simulink model "LAB1_3_mot"  (R2024b)
settings: Solver=ode3  StartTime=0.0  StopTime=10  FixedStep=0.001  RelTol=1e-3
values from neighbouring files (symbols this model uses):
  delta_c = 1/sqrt(2)    [LAB1_Corretto.m]    (also in LAB1_GIOI.m)
  K_g = K_e(2:3)    [LAB1_Corretto.m]    (also in LAB1_GIOI.m)
  KI = K_e(1)    [LAB1_Corretto.m]    (also in LAB1_GIOI.m)
  Nu = N(3)    [LAB1_Corretto.m]    (also in LAB1_GIOI.m)
  Nx = N(1:2)    [LAB1_Corretto.m]    (also in LAB1_GIOI.m)
  w_c = 2*pi*50    (= 314.159265359)    [LAB1_Corretto.m]    (also in LAB1_GIOI.m)
undefined symbols (not defined in the file or in its folder): degs2rpm, den_Hi, den_Hw, mot, National_Instruments, num_Hi, num_Hw, PCI, rpm2rads, sens
libraries: sldrtlib x3
settings Model: SimulationMode=external  ExtModeTrigDuration=100001  Creator=delpratogi  LastModifiedBy=delpratogi
settings DataIOCC: ReturnWorkspaceOutputs=off
settings HardwareCC: ProdBitPerLong=64  ProdHWDeviceType=Intel->x86-64 (Linux 64)
settings RTWCC: Description=Simulink Desktop Real-Time  SystemTargetFile=sldrt.tlc  TemplateMakefile=sldrt.tmf  RTWCompilerOptimization=on
settings CodeAppCC: MaxIdLength=95
settings SimulinkDesktopRealTimeCC: TargetLibSuffix=_sldrt.a  TargetPreCompLibLocation=C:\Program Files\MATLAB\R2024b\toolbox\sldrt\lib\win64  ParMdlRefBuildCompliant=on

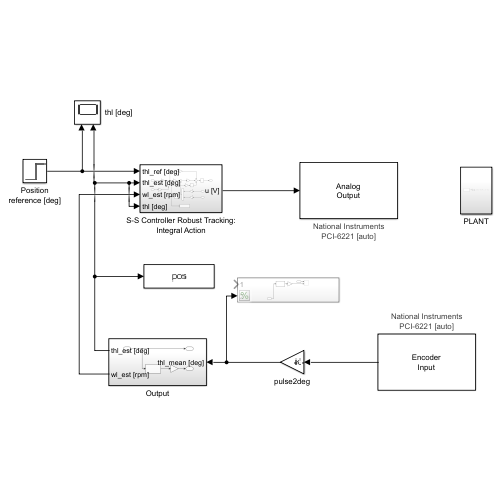
[thumbnail: Simulink's stored preview of the top-level diagram]
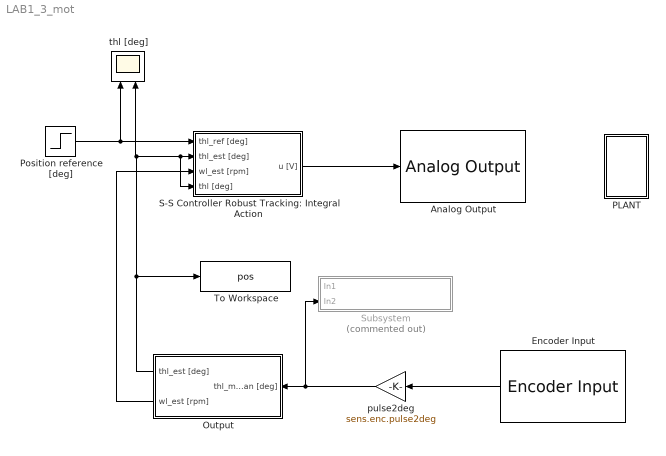
== system LAB1_3_mot ==
  Analog Output : sldrtlib/Analog Output  SampleTime=0.001  MaxMissedTicks=10  ShowMissedTicks=off  YieldWhenWaiting=off  DrvName=National_Instruments/PCI-6221  DrvAddress=4294967295  DrvOptions=[0 0 0 2 0]  Channels=1  RangeMode=1  VoltRange=1  InitialValue=0  FinalValue=0
      settings: AttributesFormatString=National Instruments\nPCI-6221 [auto]
  Encoder Input : sldrtlib/Encoder Input  SampleTime=0.001  MaxMissedTicks=10  ShowMissedTicks=off  YieldWhenWaiting=off  DrvName=National_Instruments/PCI-6221  DrvAddress=4294967295  DrvOptions=[0 0 0 2 0]  Channels=1  QuadMode=3  IndexPulse=1  InputFilter=Inf  DataType=1
      settings: AttributesFormatString=National Instruments\nPCI-6221 [auto]
  Output : Subsystem
  PLANT : Subsystem
  Position reference [deg] : Step  Time=0  After=120  SampleTime=0  ZeroCross=off
  S-S Controller Robust Tracking: Integral Action : Subsystem
  Subsystem : Subsystem  Commented=on
  To Workspace : ToWorkspace  VariableName=pos  SaveFormat=Structure With Time  SampleTime=-1
  pulse2deg : Gain  Gain=sens.enc.pulse2deg
  thl [deg] : Scope  NumInputPorts=2
  wires:
  Encoder Input/1 -> pulse2deg/1
  pulse2deg/1 -> Subsystem/2(In2), Output/1(thl_mean [deg])
  S-S Controller Robust Tracking: Integral Action/1(u [V]) -> Analog Output/1
  Output/2(wl_est [rpm]) -> S-S Controller Robust Tracking: Integral Action/3(wl_est [rpm])
  Position reference [deg]/1 -> S-S Controller Robust Tracking: Integral Action/1(thl_ref [deg]), thl [deg]/1
  Output/1(thl_est [deg]) -> S-S Controller Robust Tracking: Integral Action/4(thl [deg]), S-S Controller Robust Tracking: Integral Action/2(thl_est [deg]), thl [deg]/2, To Workspace/1

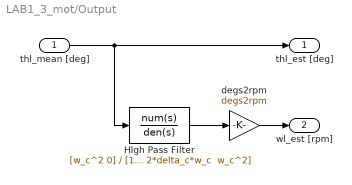
== system LAB1_3_mot/Output ==
  thl_mean [deg] : Inport
  HIgh Pass Filter : TransferFcn  Numerator=[w_c^2 0]  Denominator="[1 2*delta_c*w_c  w_c^2]"
  degs2rpm : Gain  Gain=degs2rpm
  thl_est [deg] : Outport
  wl_est [rpm] : Outport  Port=2
  wires:
  thl_mean [deg]/1 -> HIgh Pass Filter/1, thl_est [deg]/1
  HIgh Pass Filter/1 -> degs2rpm/1
  degs2rpm/1 -> wl_est [rpm]/1

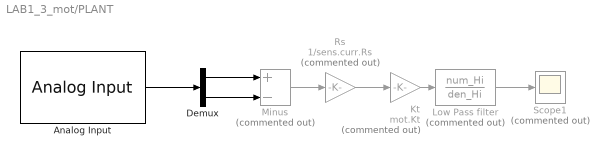
== system LAB1_3_mot/PLANT ==
  Analog Input : sldrtlib/Analog Input  SampleTime=0.001  MaxMissedTicks=10  ShowMissedTicks=off  YieldWhenWaiting=off  DrvName=National_Instruments/PCI-6221  DrvAddress=4294967295  DrvOptions=[0 0 0 2 0]  Channels=[1,2]  RangeMode=1  VoltRange=1  DataType=1
      settings: AttributesFormatString=National Instruments\nPCI-6221 [auto]
  Demux : Demux  Outputs=2
  Kt : Gain  Commented=on  Gain=mot.Kt
  Low Pass filter : TransferFcn  Commented=on  Numerator=num_Hi  Denominator=den_Hi
  Minus : Sum  Commented=on  Inputs=+-
  Rs : Gain  Commented=on  Gain=1/sens.curr.Rs
  Scope1 : Scope  Commented=on
  wires:
  Low Pass filter/1 -> Scope1/1
  Demux/1 -> Minus/1
  Minus/1 -> Rs/1
  Analog Input/1 -> Demux/1
  Kt/1 -> Low Pass filter/1
  Demux/2 -> Minus/2
  Rs/1 -> Kt/1

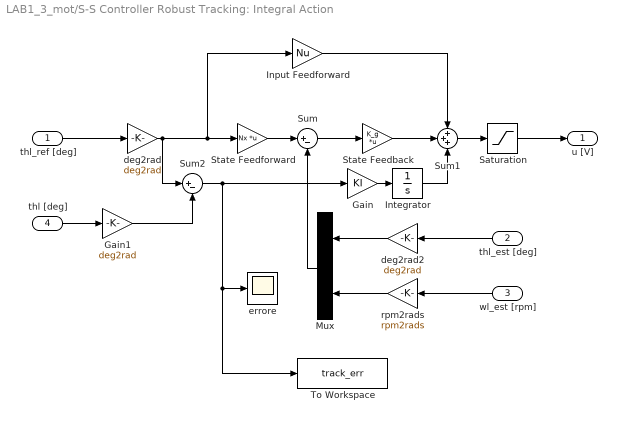
== system LAB1_3_mot/S-S Controller Robust Tracking: Integral Action ==
  thl_ref [deg] : Inport
  thl_est [deg] : Inport  Port=2
  wl_est [rpm] : Inport  Port=3
  thl [deg] : Inport  Port=4
  Gain : Gain  Gain=KI
  Gain1 : Gain  Gain=deg2rad
  Input Feedforward : Gain  Gain=Nu
  Integrator : Integrator
  Mux : Mux  Inputs=2
  Saturation : Saturate  UpperLimit=10  LowerLimit=-10  ZeroCross=off
  State Feedback : Gain  Gain=K_g  Multiplication=Matrix(K*u)
  State Feedforward : Gain  Gain=Nx  Multiplication=Matrix(K*u)
  Sum : Sum  Inputs=|+-
  Sum1 : Sum  Inputs=+++
  Sum2 : Sum  Inputs=|+-
  To Workspace : ToWorkspace  VariableName=track_err  SaveFormat=Structure With Time  SampleTime=-1
  deg2rad : Gain  Gain=deg2rad
  deg2rad2 : Gain  Gain=deg2rad
  errore : Scope
  rpm2rads : Gain  Gain=rpm2rads
  u [V] : Outport
  wires:
  Saturation/1 -> u [V]/1
  wl_est [rpm]/1 -> rpm2rads/1
  thl_ref [deg]/1 -> deg2rad/1
  Sum1/1 -> Saturation/1
  deg2rad/1 -> Sum2/1, Input Feedforward/1, State Feedforward/1
  Mux/1 -> Sum/2
  Input Feedforward/1 -> Sum1/1
  Sum/1 -> State Feedback/1
  State Feedforward/1 -> Sum/1
  rpm2rads/1 -> Mux/2
  thl_est [deg]/1 -> deg2rad2/1
  deg2rad2/1 -> Mux/1
  State Feedback/1 -> Sum1/2
  Gain/1 -> Integrator/1
  Integrator/1 -> Sum1/3
  thl [deg]/1 -> Gain1/1
  Gain1/1 -> Sum2/2
  Sum2/1 -> To Workspace/1, errore/1, Gain/1

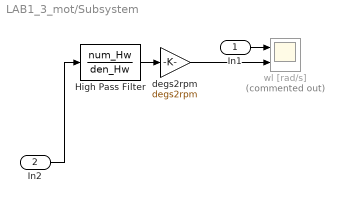
== system LAB1_3_mot/Subsystem ==
  In1 : Inport
  In2 : Inport  Port=2
  High Pass Filter : TransferFcn  Numerator=num_Hw  Denominator=den_Hw
  degs2rpm : Gain  Gain=degs2rpm
  wl [rad/s] : Scope  Commented=on  NumInputPorts=2
  wires:
  In2/1 -> High Pass Filter/1
  High Pass Filter/1 -> degs2rpm/1
  degs2rpm/1 -> wl [rad/s]/2
  In1/1 -> wl [rad/s]/1
